simulink model "lookupTableDynamic_TestGen7"  (R2017b)
settings: Solver=FixedStepDiscrete  StartTime=0.0  StopTime=10.0  RelTol=1e-3
libraries: simulink x1
settings Model: Creator=ktrinh  LastModifiedBy=ktrinh
settings DebuggingCC: ParameterOverflowMsg=none

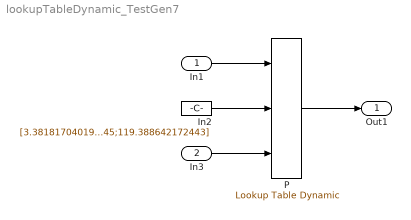
== system lookupTableDynamic_TestGen7 ==
  In1 : Inport  OutMin=1.3818  OutMax=121  OutDataTypeStr=int32  PortDimensions=[2,3]
  In3 : Inport  Port=2  PortDimensions=5
  In2 : Constant  Value=[3.38181704019352;23.284130069955;28.9082639652831;76.3817286056245;119.388642172443]  OutDataTypeStr=int32
  P : simulink/Lookup Tables/Lookup Table Dynamic  LookUpMeth=Interpolation-Extrapolation  OutDataType=fixdt('int32')  OutScaling=[]  OutputDataTypeScalingMode=Specify via dialog  OutDataTypeStr=int32  RndMeth=Ceiling  DoSatur=on
      settings: SourceProductName=Simulink
  Out1 : Outport
  wires:
  In1/1 -> P/1
  In2/1 -> P/2
  In3/1 -> P/3
  P/1 -> Out1/1
